simulink model "mavlink_missions"  (Simulink 7.8)
settings: Solver=FixedStepDiscrete  SolverMode=SingleTasking  StartTime=0.0  StopTime=10.0  FixedStep=0.01  RelTol=1e-3
InitFcn:
  | clear all
  | boat_constants
undefined symbols (not defined in the file): cpInitCommunications, Init_Reset, InitialPoint, IPStar, ISA_g, m1, m2, m3, m4, m5, m6, MavLinkInit, MavLinkReceive, MavLinkSendHeartbeat, MavLinkSendStatus, MaxDwnPthStar, switchDistance, tanIntercept, TStar, Turn2Track
libraries: uSimLib x15, dsPICdrivers x8, simulink x1
settings Model: Creator=Bryant  LastModifiedBy=Bryant
settings OptimizationCC: InlineParams=on  InlineInvariantSignals=on  PassReuseOutputArgsAs=Individual arguments  ZeroExternalMemoryAtStartup=off  ZeroInternalMemoryAtStartup=off  InitFltsAndDblsToZero=on  NoFixptDivByZeroProtection=on  EfficientFloat2IntCast=on  OptimizeModelRefInitCode=on  LifeSpan=1
settings DebuggingCC: UnderspecifiedInitializationDetection=Simplified  UniqueDataStoreMsg=error  AssertControl=DisableAll  StrictBusMsg=ErrorOnBusTreatedAsVector
settings HardwareCC: ProdBitPerInt=16  ProdBitPerPointer=16  ProdEndianess=LittleEndian  ProdWordSize=16  ProdHWDeviceType=16-bit Generic
settings SFSimCC: SimParseCustomCode=off
settings RTWCC: SystemTargetFile=dspic.tlc  MakeCommand=make_CreateMPLAB  TemplateMakefile=dspic_pic30_gcc.tmf  PostCodeGenCommand=dsPIC_Compile()  Description=Embedded Target for Microchip dsPIC (real-time)  ProcessScript=dspic_make_rtw_hook
settings RTWCC: CustomInclude=|
  | ../../mavlink
  | ../../clib
settings RTWCC: CustomSource=|
  | ../../clib/mavlink.c
  | ../../clib/uart1.c
  | ../../clib/uart2.c
  | ../../clib/Rudder.c
  | ../../clib/nmea0183.c
  | ../../clib/conversions.c
  | ../../clib/gps.c
  | ../../clib/commProtocol.c
  | ../../clib/CircularBuffer.c
settings CodeAppCC: IgnoreCustomStorageClasses=off  IgnoreTestpoints=on
settings STFCustomTargetCC: IncludeMdlTerminateFcn=off  GeneratePreprocessorConditionals=Use local settings  CombineOutputUpdateFcns=on  SuppressErrorStatus=on  ERTCustomFileBanners=on  SupportContinuousTime=off  SupportNonInlinedSFcns=off  SystemTargetFile=dspic.tlc
settings ERTTargetCC: MultiwordLength=2048  ParMdlRefBuildCompliant=off  CompOptLevelCompliant=off  ConcurrentExecutionCompliant=off  IncludeMdlTerminateFcn=off  SuppressErrorStatus=on  ERTFirstTimeCompliant=off  ModelStepFunctionPrototypeControlCompliant=off  CPPClassGenCompliant=off  ExtModeMexFile=ext_serial_win32_comm  ERTSrcFileBannerTemplate=dsPIC_code_template.cgt  ERTHdrFileBannerTemplate=dsPIC_code_template.cgt  ERTDataSrcFileTemplate=dsPIC_code_template.cgt  ERTDataHdrFileTemplate=dsPIC_code_template.cgt  ERTCustomFileTemplate=dsPIC_main.tlc  ConvertIfToSwitch=off  SuppressUnreachableDefaultCases=off
settings CustomProperty: DataType=string  Value=C:\PROGRA~1\MATLAB\R2011b\bin\win64\gmake

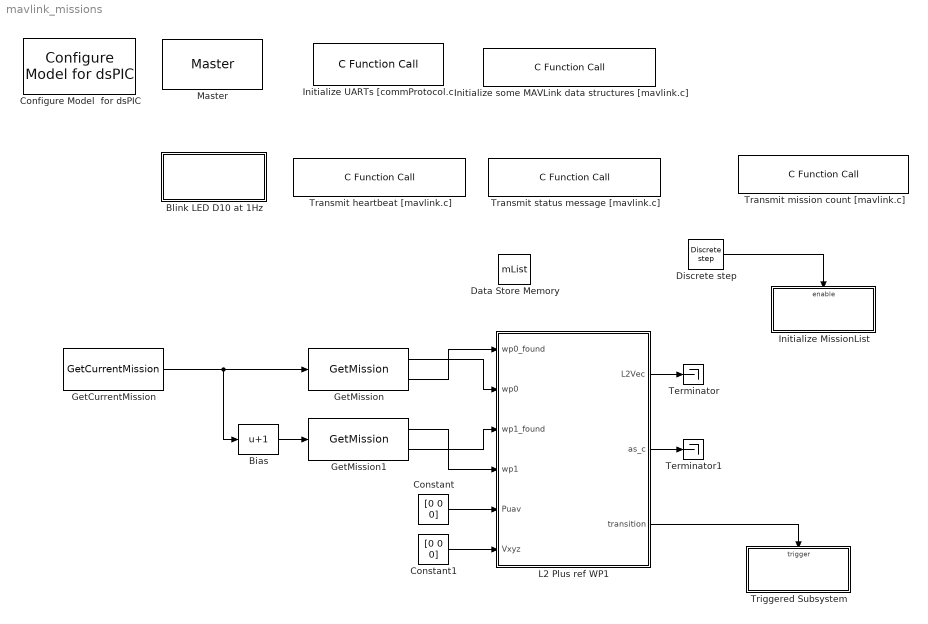
== system mavlink_missions ==
  Bias : Bias  Bias=1
  Blink LED D10 at 1Hz : Subsystem
      mask Display: disp('blink');
  Configure Model  for dsPIC : dsPICdrivers/Simulink Configuration/Configure Model  for dsPIC
  Constant : Constant  Value=[0 0 0]  OutDataTypeStr=single
  Constant1 : Constant  Value=[0 0 0]  OutDataTypeStr=single
  Data Store Memory : DataStoreMemory  DataStoreName=mList  ReadBeforeWriteMsg=warning  WriteAfterWriteMsg=warning  WriteAfterReadMsg=warning  OutDataTypeStr=Bus: MissionList
      settings: RTWStateStorageClass=ExportedGlobal
  Discrete step : uSimLib/Sources/Discrete step  start_value=1  end_value=0  transition_time=1
  GetCurrentMission : uSimLib/Mission Manager/GetCurrentMission  sampleTime=T_step
  GetMission : uSimLib/Mission Manager/GetMission  sampleTime=T_step
  GetMission1 : uSimLib/Mission Manager/GetMission  sampleTime=T_step
  Initialize MissionList : Subsystem  TreatAsAtomicUnit=on
  Initialize UARTs [commProtocol.c] : dsPICdrivers/OTHERS/C Function Call  Tag=dsPIC_dsPIC_CFunctionCall  FctUpdate=None  fctName=cpInitCommunications  INPUT_SIZE=1  INPUT1=--  INPUT2=--  INPUT3=--  OUTPUT_SIZE=1  OUTPUT1=--  SampleTime=Inf  InputType=[]  OutputType=[]  FctDeclaration=extern void cpInitCommunications();  FctCall=cpInitCommunications();  OrderingInOutPopup=None  FctStart=Start Function (Call once and only once)  FctStart_Name=cpInitCommunications  FctStart_Declaration=inline extern void cpInitCommunications();  FctStart_Call=cpInitCommunications();  FctInit=None  FctInit_Name=Init_Reset  FctInit_Declaration=inline extern void Init_Reset();  FctInit_Call=Init_Reset();  PinDigitalInput=[]  PinDigitalOutput=[]  AnalogueInput=[]
  Initialize some MAVLink data structures [mavlink.c] : dsPICdrivers/OTHERS/C Function Call  Tag=dsPIC_dsPIC_CFunctionCall  FctUpdate=None  fctName=MavLinkSendHeartbeat  INPUT_SIZE=1  INPUT1=--  INPUT2=--  INPUT3=--  OUTPUT_SIZE=1  OUTPUT1=--  SampleTime=1  InputType=[]  OutputType=[]  FctDeclaration=extern void MavLinkSendHeartbeat();  FctCall=MavLinkSendHeartbeat();  OrderingInOutPopup=None  FctStart=Start Function (Call once and only once)  FctStart_Name=MavLinkInit  FctStart_Declaration=inline extern void MavLinkInit();  FctStart_Call=MavLinkInit();  FctInit=None  FctInit_Name=Init_Reset  FctInit_Declaration=inline extern void Init_Reset();  FctInit_Call=Init_Reset();  PinDigitalInput=[]  PinDigitalOutput=[]  AnalogueInput=[]
  L2 Plus ref WP1 : MATLAB Function  TreatAsAtomicUnit=on
  Master : dsPICdrivers/Master  Tag=dsPIC_MASTER  Priority=1  TimeStepType=Timer1  picType=33fJ256GP710A  fcy=40000000  Quartz_33f=8e6  PLLActive_33f=on  fcyDesired_33f=40000000  tmr1="[8  49999  0]"  tmr1Info="Time Step : 0.01  ;   Error : 0%  PR1=49999"  tmr2345="[0  0  0  0  0  0  0  0]"  tmr2345cfg=[-1 -1 -1 -1 -1 -1 -1 -1]  IOautoConf=on  typePort="[ 0   0   0   0   0   0   0  10   0   0   0   0   0   0   0   0   0   0   0   0   0   0   0   0   0   0   0   0   0   0   0   0   0   0   0   0   0   0   0   0   0   0   0   0   0   0   0   0   0   0   0   0   0   0   0   0   0   0   0   0   0   0   0   0   0   0   0   0   0   0   0   0   0   0   0   0   0   0   0   0   0   0   0   0   0   0   0   0   0   0   0   0   0   0   0   0   0   0   0   0   0   0   0   0   0   0   0   0   0   0   0   0 ]"  TRIS="[ 65407  65535  65535  65535  65535  65535  65535 ]"  ADPCFG=8388608  MasterBusyPort=None  MasterOverloadPort=None  FOSC=Quartz (XT - HS)  ClockSwitchMonitor=Both disabled  TempProtection_33f=TEMP_ON  FPBOR=<empty>  PWRT=disable  MCLR=<empty>  ICD=ICS_PGD1  JTAGEN=JTAGEN_OFF  PowerSave=off  OverrideFcy=off  NewFcy=1e6  PR2345="[65535  65535  65535  65535  65535  65535  65535  65535]"
  Terminator : Terminator
  Terminator1 : Terminator
  Transmit heartbeat [mavlink.c] : dsPICdrivers/OTHERS/C Function Call  Tag=dsPIC_dsPIC_CFunctionCall  FctUpdate=Output Function  fctName=MavLinkSendHeartbeat  INPUT_SIZE=1  INPUT1=--  INPUT2=--  INPUT3=--  OUTPUT_SIZE=1  OUTPUT1=--  SampleTime=1  InputType=[ ]  OutputType=[ ]  FctDeclaration=extern void MavLinkSendHeartbeat();  FctCall=MavLinkSendHeartbeat();  OrderingInOutPopup=None  FctStart=None  FctStart_Name=cpInitCommunications  FctStart_Declaration=inline extern void cpInitCommunications();  FctStart_Call=cpInitCommunications();  FctInit=None  FctInit_Name=Init_Reset  FctInit_Declaration=inline extern void Init_Reset();  FctInit_Call=Init_Reset();  PinDigitalInput=[]  PinDigitalOutput=[]  AnalogueInput=[]
  Transmit mission count [mavlink.c] : dsPICdrivers/OTHERS/C Function Call  Tag=dsPIC_dsPIC_CFunctionCall  FctUpdate=Output Function  fctName=MavLinkReceive  INPUT_SIZE=1  INPUT1=--  INPUT2=--  INPUT3=--  OUTPUT_SIZE=1  OUTPUT1=--  SampleTime=.01  InputType=[ ]  OutputType=[ ]  FctDeclaration=extern void MavLinkReceive();  FctCall=MavLinkReceive();  OrderingInOutPopup=None  FctStart=None  FctStart_Name=cpInitCommunications  FctStart_Declaration=inline extern void cpInitCommunications();  FctStart_Call=cpInitCommunications();  FctInit=None  FctInit_Name=Init_Reset  FctInit_Declaration=inline extern void Init_Reset();  FctInit_Call=Init_Reset();  PinDigitalInput=[]  PinDigitalOutput=[]  AnalogueInput=[]
  Transmit status message [mavlink.c] : dsPICdrivers/OTHERS/C Function Call  Tag=dsPIC_dsPIC_CFunctionCall  FctUpdate=Output Function  fctName=MavLinkSendStatus  INPUT_SIZE=1  INPUT1=--  INPUT2=--  INPUT3=--  OUTPUT_SIZE=1  OUTPUT1=--  SampleTime=1  InputType=[ ]  OutputType=[ ]  FctDeclaration=extern void MavLinkSendStatus();  FctCall=MavLinkSendStatus();  OrderingInOutPopup=None  FctStart=None  FctStart_Name=cpInitCommunications  FctStart_Declaration=inline extern void cpInitCommunications();  FctStart_Call=cpInitCommunications();  FctInit=None  FctInit_Name=Init_Reset  FctInit_Declaration=inline extern void Init_Reset();  FctInit_Call=Init_Reset();  PinDigitalInput=[]  PinDigitalOutput=[]  AnalogueInput=[]
  Triggered Subsystem : Subsystem  TreatAsAtomicUnit=on
  wires:
  Discrete step/1 -> Initialize MissionList/Enable
  GetCurrentMission/1 -> GetMission/1, Bias/1
  GetMission/2 -> L2 Plus ref WP1/1(wp0_found)
  GetMission/1 -> L2 Plus ref WP1/2(wp0)
  GetMission1/1 -> L2 Plus ref WP1/4(wp1)
  GetMission1/2 -> L2 Plus ref WP1/3(wp1_found)
  Bias/1 -> GetMission1/1
  Constant/1 -> L2 Plus ref WP1/5(Puav)
  Constant1/1 -> L2 Plus ref WP1/6(Vxyz)
  L2 Plus ref WP1/3(transition) -> Triggered Subsystem/Trigger
  L2 Plus ref WP1/1(L2Vec) -> Terminator/1
  L2 Plus ref WP1/2(as_c) -> Terminator1/1

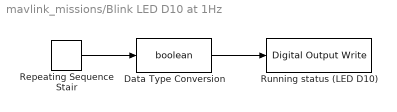
== system mavlink_missions/Blink LED D10 at 1Hz ==
  Data Type Conversion : DataTypeConversion  OutDataTypeStr=boolean  RndMeth=Simplest
  Repeating Sequence Stair : simulink/Sources/Repeating Sequence Stair  OutValues=[1 0]  tsamp=1  OutMin=[]  OutMax=[]  OutDataTypeStr=double  OutputDataTypeScalingMode=double  OutDataType=fixdt(0,8)  ConRadixGroup=Best Precision: Vector-wise  OutScaling=2^-12
  Running status (LED D10) : dsPICdrivers/Digital I//O/Digital Output Write  Tag=dsPIC_Digital_Output  Priority=5  PORT=A  Pin=[7]  Simultaneous=off  OrderingInOutPopup=None
  wires:
  Repeating Sequence Stair/1 -> Data Type Conversion/1
  Data Type Conversion/1 -> Running status (LED D10)/1

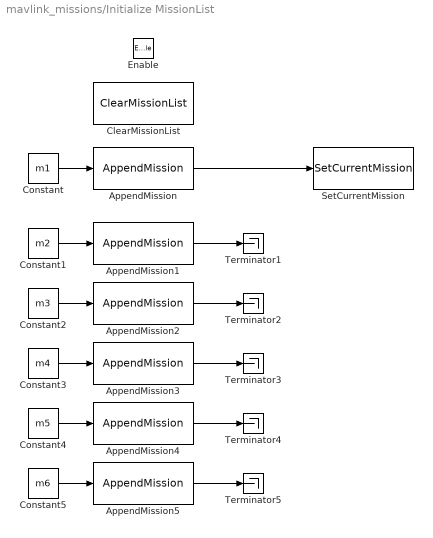
== system mavlink_missions/Initialize MissionList ==
  Enable : EnablePort
  AppendMission{,1..5} (6 alike) : uSimLib/Mission Manager/AppendMission  sampleTime=T_step
  ClearMissionList : uSimLib/Mission Manager/ClearMissionList  Priority=1  SystemSampleTime=-1
  Constant : Constant  Value=m1  OutDataTypeStr=Bus: Mission
  Constant1 : Constant  Value=m2  OutDataTypeStr=Bus: Mission
  Constant2 : Constant  Value=m3  OutDataTypeStr=Bus: Mission
  Constant3 : Constant  Value=m4  OutDataTypeStr=Bus: Mission
  Constant4 : Constant  Value=m5  OutDataTypeStr=Bus: Mission
  Constant5 : Constant  Value=m6  OutDataTypeStr=Bus: Mission
  SetCurrentMission : uSimLib/Mission Manager/SetCurrentMission  sampleTime=-1
  Terminator{1..5} (5 alike) : Terminator
  wires:
  AppendMission/1 -> SetCurrentMission/1
  Constant/1 -> AppendMission/1
  AppendMission1/1 -> Terminator1/1
  Constant1/1 -> AppendMission1/1
  AppendMission2/1 -> Terminator2/1
  Constant2/1 -> AppendMission2/1
  AppendMission3/1 -> Terminator3/1
  Constant3/1 -> AppendMission3/1
  AppendMission4/1 -> Terminator4/1
  Constant4/1 -> AppendMission4/1
  AppendMission5/1 -> Terminator5/1
  Constant5/1 -> AppendMission5/1

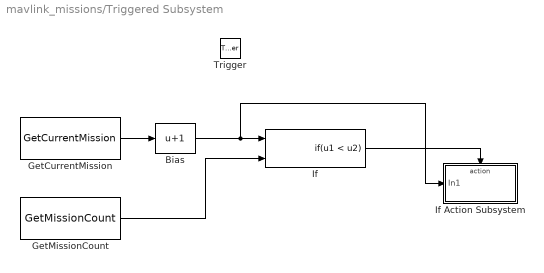
== system mavlink_missions/Triggered Subsystem ==
  Trigger : TriggerPort
  Bias : Bias  Bias=1
  GetCurrentMission : uSimLib/Mission Manager/GetCurrentMission  sampleTime=-1
  GetMissionCount : uSimLib/Mission Manager/GetMissionCount  sampleTime=-1
  If : If  NumInputs=2  IfExpression=u1 < u2  ShowElse=off
  If Action Subsystem : Subsystem  TreatAsAtomicUnit=on
  wires:
  GetCurrentMission/1 -> Bias/1
  GetMissionCount/1 -> If/2
  Bias/1 -> If Action Subsystem/1(In1), If/1
  If/1 -> If Action Subsystem/Action

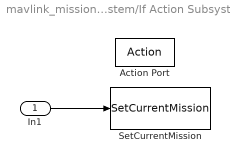
== system mavlink_missions/Triggered Subsystem/If Action Subsystem ==
  In1 : Inport
  Action Port : ActionPort  ActionType=then
  SetCurrentMission : uSimLib/Mission Manager/SetCurrentMission  sampleTime=-1
  wires:
  In1/1 -> SetCurrentMission/1

== matlab function L2 Plus ref WP1 ==
  data: wp0_found input boolean; wp0 input Bus: Mission size=1; wp1_found input boolean; wp1 input Bus: Mission size=1; L2Vec output single; Puav input single size=3; Vxyz input single size=3; switchDistance parameter double size=1; ISA_g parameter double; tanIntercept parameter double; MaxDwnPthStar parameter double; Turn2Track parameter double; InitialPoint parameter double; IPStar parameter double; TStar parameter double; as_c output single; transition output boolean
function [L2Vec, as_c, transition] = L2PlusWP1(wp0_found, wp0, wp1_found, wp1, Puav, Vxyz, switchDistance, ...
    ISA_g, tanIntercept, MaxDwnPthStar,Turn2Track,...
    InitialPoint, IPStar, TStar)
%==============================
%     computes bank angle command for following a straight line
%     by creating an aim point that may be more than L2 away 
%     from the UAV. The aim point is (usually) farther along the path 
%     toward WP1 than the UAV, and the intercept
%     angle is less than or equal to a specified value. This limits the intercept
%     angle even when the UAV is within L2 of the path.
%     See L2PlusWP1.m for details
%
%         INPUTS   
%             T1      unit vector WP0-->WP1
%             N1      normal to T1
%             wp0     Mission bus with the from mission data in it
%             wp1     Mission bus with the to/current mission data in it
%             Puav    position of UAV
%             Vxyz    Inertial velocity
%             switchDistance distance from WP1 to switch to WP2
%
%         PARAMETERS
%             ISA_g   gravity
%             tanIntercept  tangent of intercept angle
%             MaxDwnPthStar L2 multiplier to determmine downpath aimpoint
%             Turn2Track    true to turn toward T1 instead of L2
%             InitialPoint  true if no line tracking at first--fly direct to some initial point
%             IPStar        L2 multiplier to determing distance of IP from first WP0
%             Tstar         was called L2Base, time constant of response
%             
%         OUTPUTS
%             L2Vec   L2 vector toward aim point
%             as_c    commanded lateral acceleration
%             transition A boolean of whether to transition or not to the next waypoint

    persistent IPActive;  %true if flying toward IP
    persistent IP; % location of initial point

    persistent direction; % Keep track of the direction for patrol mode
    if isempty(direction)
        direction = int8(1);
    end
    
    Pwp1 = single(zeros(3,1));
    Pe_y = single(0);
    Dist2WP1 = single(0);
    MinDownPath = single(0);
    Dist2WPSwitch = single(0);
    L2DownPath = single(0);
    L2ToT = single(zeros(3,1));
    L2Vec = single(zeros(3,1));
    IP1 = single([0; 0;-999]); %signal for no IP
    as_c = single(0);
    transition = false;
    
    Pne = [Puav(1); Puav(2); 0]; %horizontal position
    Vne = [Vxyz(1); Vxyz(2); 0]; % horizontal velocity
    Groundspeed = norm(Vne);
    L2 = single(TStar*Groundspeed);
    
    WP0 = wp0.coordinates;
    WP1 = wp1.coordinates;
    
    if ~wp0_found || ~wp1_found
        return;
    end
    % Calculate N1 and T1
    assert(norm(WP1 - WP0) ~= 0);
    T1 = WP1 - WP0;
    T1 = T1/norm(T1);
    N1 = [-T1(2); T1(1); 0];
    
%     initialize the initial point
    if (isempty(IPActive))
        if (InitialPoint)
%             IP is set relative to the first "from" waypoint
            IPActive = -1;
            IP = [WP0(1); WP0(2); 0] - L2*IPStar*T1;
            
            if (norm(IP-Pne) < .001)
                IPActive = 0;
                IP = single([0; 0; -999]);
            end
        else
            IPActive = 0;
            IP = single([0; 0;-999]); %signal for no IP
        end
    end
    IP1 = IP;
    
    
    if (IPActive)
%         no line tracking, direct to IP
        L2Vec = L2*(IP - Pne)/norm(IP - Pne);
%         check to see if at the IP to terminate this mode
        if norm(IP - Pne) < .1*L2
            IPActive = 0;
        end
    else
         if (Pne(1) < 2)
             IP1 = IP1;
         end
%         IP not active, track WP lines
        Pwp1 = Pne - [WP1(1); WP1(2); 0]; % position of UAV relative to WP1
        Pe_y = single(Pwp1'*N1); % cross track error
        Dist2WP1 = -single(Pwp1'*T1); % distance to WP1

%         minimum down path distance for Aim Point intersection on T
%         is determined by the intercept angle but limited 
%         in case of very distant intecepts to MaxDwnPthStar*L2
        MinDownPath = single ( min( abs(Pe_y)/tanIntercept, MaxDwnPthStar*L2)); 
        Dist2WPSwitch = Dist2WP1 - switchDistance;
        if ( abs(Pe_y) > L2 )
    %             Make sure aimpoint is no closer to waypoint than calculated switch point.
            L2DownPath = MinDownPath;
        else
    %             within L2 of T and Dist2WPSwitch >= 0, but limit angle of L2 wrt T
            L2DownPath = (max(MinDownPath, (sqrt( L2^2 - Pe_y^2 ))));
        end
        
        if ( Dist2WPSwitch < 0 )
            transition = true;
        end
        
         % vector from Pwp1 to aim point on T1
         L2ToT = single(( Dist2WP1 - L2DownPath )*(-T1) - Pwp1);
         if (norm(L2ToT) < .001)
             L2Vec = L2*T1;
         else
            L2Vec = single(L2*( L2ToT/norm(L2ToT) )); % limit size to L2
         end
    %         L2Vec = L2ToT;
%         dummy statements
    end
    Zprod = single(Vxyz(1)*L2Vec(2) - Vxyz(2)*L2Vec(1)); %Z component of cross product
    sinEta = single(Zprod/(Groundspeed*L2));

    as_c = single(2*Groundspeed^2/(L2)*sinEta);

%         now override bank angle if heading in the wrong direction
    if ( Turn2Track && Dist2WPSwitch > 0 && ~IPActive ) 
%             turn to track not L2, gives min displacement from track
        if ( T1'*Vxyz < 0 )
            if ( Pe_y > 0 )
                as_c = single(99);
            else
                as_c = single(-99);
            end
        end
     else
%           turn toward L2, give min displacement toward WP0
        if ( L2Vec'*Vxyz < 0 )
            if ( sinEta < 0 )
                as_c = single(-99);
            else
                as_c = single(99);
            end
        end
    end
end
